simulink library "wbme_lib"  (R2018b)
settings: Solver=VariableStepAuto  StartTime=0.0  StopTime=10.0  RelTol=1e-3
undefined symbols (not defined in the file or in its folder): DiscIntNeverNeededParam, WBMO, WBMO_notune
settings Model: Creator=Ybeyer  LastModifiedBy=yannic
settings DebuggingCC: LibraryContextMissingDiagnostic=none
settings SFSimCC: SimUseLocalCustomCode=off
settings RTWCC: RTWUseLocalCustomCode=off
settings CodeAppCC: StateflowObjectComments=on

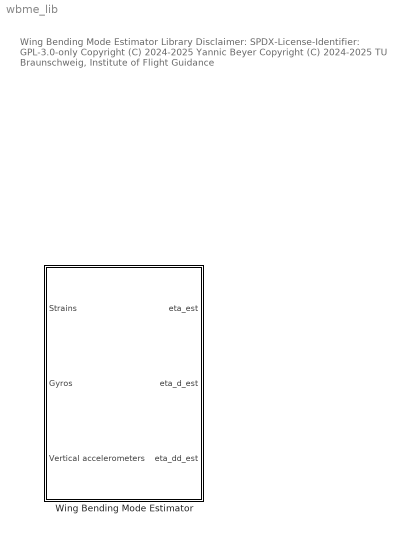
== system wbme_lib ==
  note: Wing Bending Mode Estimator Library
      |
      | Disclaimer:
      | SPDX-License-Identifier: GPL-3.0-only
      |
      | Copyright (C) 2024-2025 Yannic Beyer
      | Copyright (C) 2024-2025 TU Braunschweig, Institute of Flight Guidance
  Wing Bending Mode Estimator : Subsystem  mask{wbmo=WBMO, wbmo_notune=WBMO_notune}
      mask prompts: wbmo "Observer tunable parameters struct, see wbmoCreate"; wbmo_notune "Observer non-tunable parameters struct, see wbmoCreate"
      mask DialogControl DescGroupVar Prompt: Wing Bending Mode Observer

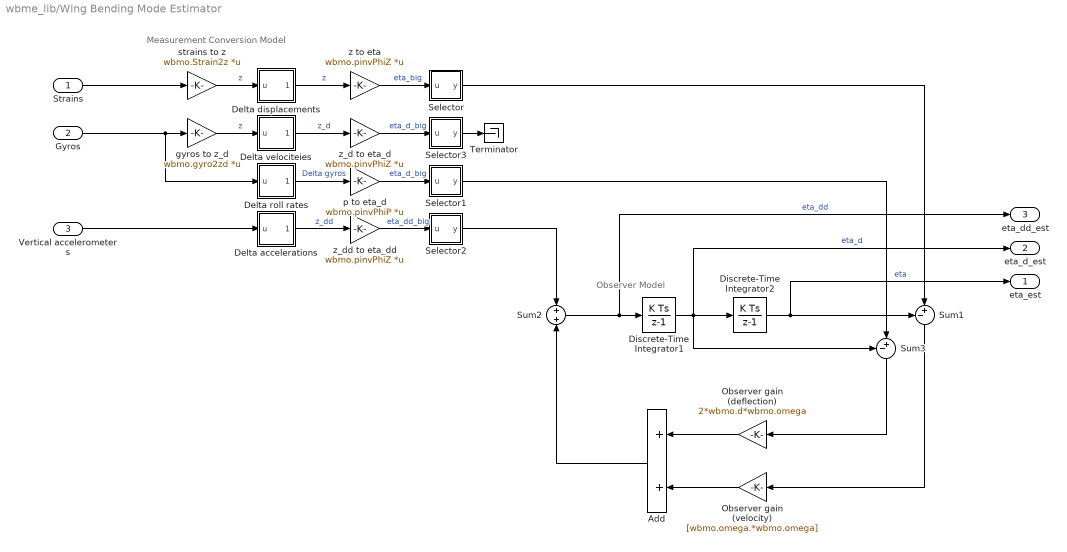
== system wbme_lib/Wing Bending Mode Estimator ==
  note: Observer Model
  note: Measurement Conversion Model
  Strains : Inport  SampleTime=wbmo_notune.sample_time
  Gyros : Inport  Port=2  SampleTime=wbmo_notune.sample_time
  Vertical accelerometers : Inport  Port=3  SampleTime=wbmo_notune.sample_time
  Add : Sum
  Delta accelerations : MATLAB Function  TreatAsAtomicUnit=on
  Delta displacements : MATLAB Function  TreatAsAtomicUnit=on
  Delta roll rates : MATLAB Function  TreatAsAtomicUnit=on
  Delta velociteies : MATLAB Function  TreatAsAtomicUnit=on
  Discrete-Time Integrator1 : DiscreteIntegrator  SampleTime=-1  ICPrevOutput=DiscIntNeverNeededParam  ICPrevScaledInput=DiscIntNeverNeededParam
  Discrete-Time Integrator2 : DiscreteIntegrator  SampleTime=-1  ICPrevOutput=DiscIntNeverNeededParam  ICPrevScaledInput=DiscIntNeverNeededParam
  Observer gain (deflection) : Gain  Gain=2*wbmo.d*wbmo.omega
  Observer gain (velocity) : Gain  Gain=[wbmo.omega.*wbmo.omega]
  Selector : Subsystem  mask{mode_shape_idx=wbmo_notune.mode_idx_obs}
      mask prompts: mode_shape_idx "Mode shape indices"
  Selector1 : Subsystem  mask{mode_shape_idx=wbmo_notune.mode_idx_obs}
      mask prompts: mode_shape_idx "Mode shape indices"
  Selector2 : Subsystem  mask{mode_shape_idx=wbmo_notune.mode_idx_obs}
      mask prompts: mode_shape_idx "Mode shape indices"
  Selector3 : Subsystem  mask{mode_shape_idx=wbmo_notune.mode_idx_obs}
      mask prompts: mode_shape_idx "Mode shape indices"
  Sum1 : Sum  Inputs=-+|
  Sum2 : Sum
  Sum3 : Sum  Inputs=-+|
  Terminator : Terminator
  gyros to z_d : Gain  Gain=wbmo.gyro2zd  Multiplication=Matrix(K*u)
  p to eta_d : Gain  Gain=wbmo.pinvPhiP  Multiplication=Matrix(K*u)
  strains to z : Gain  Gain=wbmo.Strain2z  Multiplication=Matrix(K*u)
  z to eta : Gain  Gain=wbmo.pinvPhiZ  Multiplication=Matrix(K*u)
  z_d to eta_d : Gain  Gain=wbmo.pinvPhiZ  Multiplication=Matrix(K*u)
  z_dd to eta_dd : Gain  Gain=wbmo.pinvPhiZ  Multiplication=Matrix(K*u)
  eta_est : Outport
  eta_d_est : Outport  Port=2
  eta_dd_est : Outport  Port=3
  wires:
  p to eta_d/1 -> Selector1/1(u)  "eta_d_big"
  z to eta/1 -> Selector/1(u)  "eta_big"
  Add/1 -> Sum2/2
  Sum2/1 -> eta_dd_est/1, Discrete-Time Integrator1/1  "eta_dd"
  z_dd to eta_dd/1 -> Selector2/1(u)  "eta_dd_big"
  Selector/1(y) -> Sum1/2
  Discrete-Time Integrator1/1 -> Sum3/1, Discrete-Time Integrator2/1, eta_d_est/1  "eta_d"
  Gyros/1 -> Delta roll rates/1(u), gyros to z_d/1
  Discrete-Time Integrator2/1 -> Sum1/1, eta_est/1  "eta"
  Sum1/1 -> Observer gain (velocity)/1
  Vertical accelerometers/1 -> Delta accelerations/1(u)
  strains to z/1 -> Delta displacements/1(u)  "z"
  Selector1/1(y) -> Sum3/2
  Selector2/1(y) -> Sum2/1
  Strains/1 -> strains to z/1
  Delta roll rates/1(Delta_u) -> p to eta_d/1  "Delta gyros"
  Delta accelerations/1(Delta_u) -> z_dd to eta_dd/1  "z_dd"
  Sum3/1 -> Observer gain (deflection)/1
  Observer gain (deflection)/1 -> Add/1
  Observer gain (velocity)/1 -> Add/2
  Delta displacements/1(Delta_u) -> z to eta/1  "z"
  gyros to z_d/1 -> Delta velociteies/1(u)  "z"
  Delta velociteies/1(Delta_u) -> z_d to eta_d/1  "z_d"
  z_d to eta_d/1 -> Selector3/1(u)  "eta_d_big"
  Selector3/1(y) -> Terminator/1

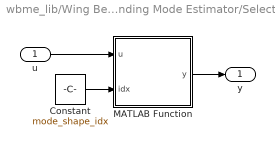
== system wbme_lib/Wing Bending Mode Estimator/Selector ==
  u : Inport
  Constant : Constant  Value=mode_shape_idx
  MATLAB Function : MATLAB Function  TreatAsAtomicUnit=on
  y : Outport
  wires:
  MATLAB Function/1(y) -> y/1
  u/1 -> MATLAB Function/1(u)
  Constant/1 -> MATLAB Function/2(idx)

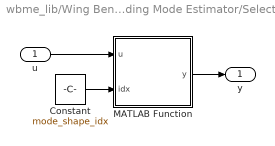
== system wbme_lib/Wing Bending Mode Estimator/Selector1 ==
  u : Inport
  Constant : Constant  Value=mode_shape_idx
  MATLAB Function : MATLAB Function  TreatAsAtomicUnit=on
  y : Outport
  wires:
  Constant/1 -> MATLAB Function/2(idx)
  u/1 -> MATLAB Function/1(u)
  MATLAB Function/1(y) -> y/1

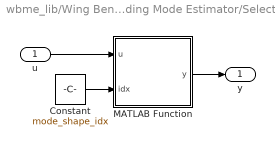
== system wbme_lib/Wing Bending Mode Estimator/Selector2 ==
  u : Inport
  Constant : Constant  Value=mode_shape_idx
  MATLAB Function : MATLAB Function  TreatAsAtomicUnit=on
  y : Outport
  wires:
  MATLAB Function/1(y) -> y/1
  u/1 -> MATLAB Function/1(u)
  Constant/1 -> MATLAB Function/2(idx)

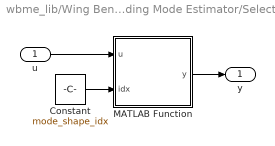
== system wbme_lib/Wing Bending Mode Estimator/Selector3 ==
  u : Inport
  Constant : Constant  Value=mode_shape_idx
  MATLAB Function : MATLAB Function  TreatAsAtomicUnit=on
  y : Outport
  wires:
  Constant/1 -> MATLAB Function/2(idx)
  u/1 -> MATLAB Function/1(u)
  MATLAB Function/1(y) -> y/1

== matlab function wbme_lib/Wing Bending Mode Estimator/Selector1/MATLAB Function ==
  data: u input; y output; idx input
function y = fcn(u, idx)
y = u(idx);
end

== matlab function wbme_lib/Wing Bending Mode Estimator/Selector/MATLAB Function ==
  data: u input; y output; idx input
function y = fcn(u, idx)
y = u(idx);
end

== matlab function wbme_lib/Wing Bending Mode Estimator/Selector2/MATLAB Function ==
  data: u input; y output; idx input
function y = fcn(u, idx)
y = u(idx);
end

== matlab function wbme_lib/Wing Bending Mode Estimator/Delta displacements ==
  data: u input; Delta_u output
function Delta_u = fcn(u)
Delta_u = zeros(length(u)-1,1);
u_center = u(end/2+0.5);
Delta_u(1:end/2) = u(1:end/2-0.5) - u_center;
Delta_u(end/2+1:end) = u(end/2+1.5:end) - u_center;
end

== matlab function wbme_lib/Wing Bending Mode Estimator/Delta velociteies ==
  data: u input; Delta_u output
function Delta_u = fcn(u)
Delta_u = zeros(length(u)-1,1);
u_center = u(end/2+0.5);
Delta_u(1:end/2) = u(1:end/2-0.5) - u_center;
Delta_u(end/2+1:end) = u(end/2+1.5:end) - u_center;
end

== matlab function wbme_lib/Wing Bending Mode Estimator/Selector3/MATLAB Function ==
  data: u input; y output; idx input
function y = fcn(u, idx)
y = u(idx);
end

== matlab function wbme_lib/Wing Bending Mode Estimator/Delta roll rates ==
  data: u input; Delta_u output
function Delta_u = fcn(u)
Delta_u = zeros(length(u)-1,1);
u_center = u(end/2+0.5);
Delta_u(1:end/2) = u(1:end/2-0.5) - u_center;
Delta_u(end/2+1:end) = u(end/2+1.5:end) - u_center;
end

== matlab function wbme_lib/Wing Bending Mode Estimator/Delta accelerations ==
  data: u input; Delta_u output
function Delta_u = fcn(u)
Delta_u = zeros(length(u)-1,1);
u_center = u(end/2+0.5);
Delta_u(1:end/2) = u(1:end/2-0.5) - u_center;
Delta_u(end/2+1:end) = u(end/2+1.5:end) - u_center;
end
